simulink model "bch"  (R2022b)
settings: Solver=VariableStepAuto  StartTime=0.0  StopTime=10  RelTol=1e-3
libraries: commblkcod2 x2
settings Model: Creator=senol  LastModifiedBy=senol
settings DebuggingCC: ParameterOverflowMsg=none  ParameterUnderflowMsg=error

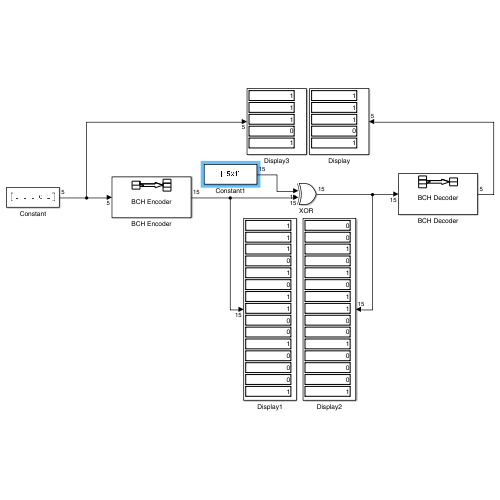
[thumbnail: Simulink's stored preview of the top-level diagram]
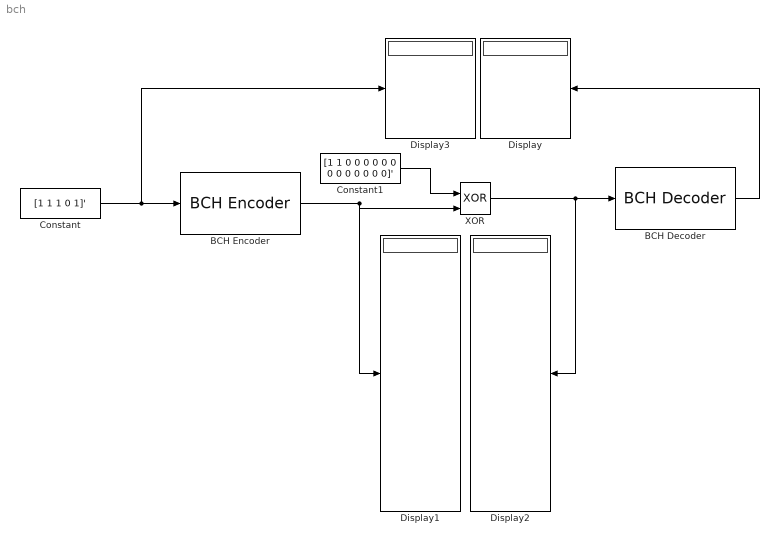
== system bch ==
  BCH Decoder : commblkcod2/BCH Decoder  n=15  k=5  specShortening=off  shortenedK=5  specGenPoly=off  genPoly='X^10 + X^8 + X^5 + X^4 + X^2 + X + 1'  specPrimPoly=off  prPoly='X^4 + X + 1'  specDisableGenCheck=off  specPuncture=off  punctVec=[ones(8,1); zeros(2,1)]  specErasurePort=off  showNumErr=off
  BCH Encoder : commblkcod2/BCH Encoder  n=15  k=5  specShortening=off  shortenedK=5  specGenPoly=off  genPoly='X^10 + X^8 + X^5 + X^4 + X^2 + X + 1'  specPrimPoly=off  prPoly='X^4 + X + 1'  specDisableGenCheck=off  specPuncture=off  punctVec=[ones(8,1); zeros(2,1)]
  Constant : Constant  Value=[1 1 1 0 1]'  OutDataTypeStr=boolean
  Constant1 : Constant  Value=[1 1 0 0 0 0 0 0 0 0 0 0 0 0 0]'  OutDataTypeStr=boolean
  Display{,1..3} (4 alike) : Display
  XOR : Logic  Operator=XOR  IconShape=distinctive  AllPortsSameDT=off  OutDataTypeStr=boolean
  wires:
  BCH Encoder/1 -> Display1/1, XOR/2
  Constant/1 -> Display3/1, BCH Encoder/1
  BCH Decoder/1 -> Display/1
  XOR/1 -> BCH Decoder/1, Display2/1
  Constant1/1 -> XOR/1
